simulink model "DataAnalysis"  (Simulink 7.6)
settings: Solver=FixedStepDiscrete  StartTime=0.0  StopTime=0  RelTol=1e-3
undefined symbols (not defined in the file or in its folder): gray, Rec, SDTV
libraries: vipconversions x2, vipsnks x1, viptextngfix x1, vipsrcs x1, viptransforms x1
settings Model: Creator=Administrator  LastModifiedBy=Administrator
settings OptimizationCC: OptimizeModelRefInitCode=on  LifeSpan=1
settings RTWCC: SystemTargetFile=ert.tlc  GenCodeOnly=on  TemplateMakefile=ert_default_tmf  Description=Real-Time Workshop Embedded Coder  GenerateReport=on  ProcessScript=ert_make_rtw_hook  IncludeHyperlinkInReport=on  LaunchReport=on  TargetLang=C++
settings CodeAppCC: IgnoreCustomStorageClasses=off
settings ERTTargetCC: MultiwordLength=2048  GenerateSampleERTMain=on  ERTCustomFileTemplate=example_file_process.tlc  ConvertIfToSwitch=off

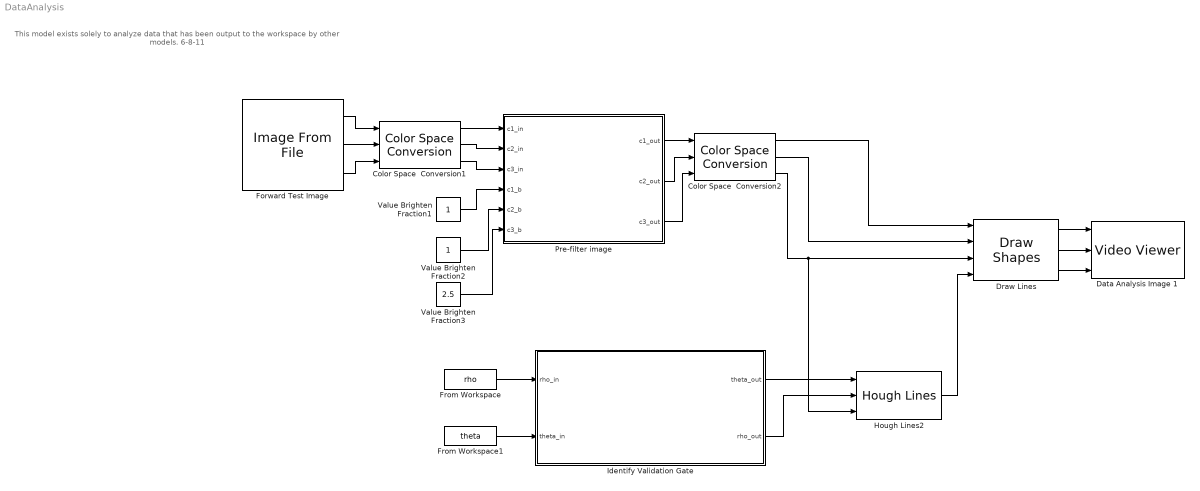
== system DataAnalysis ==
  note: This model exists solely to analyze
      | data that has been output to the
      | workspace by other models.
      |
      | 6-8-11
  Color Space  Conversion1 : vipconversions/Color Space  Conversion  conversion=Obsolete  conversionActive=R'G'B' to HSV  wp_str=D50  rec=Rec. 601 (SDTV)  sys=1125/60/2:1  imagePorts=Separate color signals
  Color Space  Conversion2 : vipconversions/Color Space  Conversion  conversion=Obsolete  conversionActive=HSV to R'G'B'  wp_str=D50  rec=Rec. 601 (SDTV)  sys=1125/60/2:1  imagePorts=Separate color signals
  Data Analysis Image 1 : vipsnks/Video Viewer  DialogControllerArgs=DataTag1  inputType=Obsolete7b  imagePorts=Separate color signals  useColorMap=off  colormapValue=gray(256)  specRange=off  minInputVal=0  maxInputVal=255  FigPos=[39 393 492 307]  AxisZoom=on  trueSizedOnce=off  OpenAtMdlStart=on
  Draw Lines : viptextngfix/Draw Shapes  DialogController=vipDDGCreate  DialogControllerArgs=DataTag2  shape=Lines  fill=off  fillClrSource=Specify via dialog  display=User-specified value  intensity=200  color=[.8 .8 .8]  opacity=0.6  viewport=Entire image  antialiasing=off  inType=Obsolete  imagePorts=Separate color signals  prodOutputMode=Binary point scaling  prodOutputWordLength=32  prodOutputFracLength=14  memoryMode=Specify word length  memoryWordLength=16  memoryFracLength=15  roundingMode=Floor  overflowMode=off
  Forward Test Image : vipsrcs/Image From File  Tag=vipblks_nd  DialogController=vipDDGCreate  DialogControllerArgs=DataTag3  SystemSampleTime=-1  FileName=C:\Documents and Settings\Administrator\My Documents\Academics\Summer 2011\AUVT\Models\Test_Models\Images\gate8.PNG  imagePorts=Separate color signals  Ts=-1  ImageDataType=double  Signed=on  WordLength=16  sdImageDataType=uint(8)  FractionLengthMode=User-defined  FractionLength=15  OutPortLabels=R|G|B
  From Workspace : FromWorkspace  VariableName=rho  SampleTime=0
  From Workspace1 : FromWorkspace  VariableName=theta  SampleTime=0
  Hough Lines2 : viptransforms/Hough Lines  DialogController=vipDDGCreate  DialogControllerArgs=DataTag4  sineCompMethod=Trigonometric function  thetaRes=pi/180  firstCoeffMode=Specify word length  firstCoeffWordLength=16  firstCoeffFracLength=15  prodOutputMode=Binary point scaling  prodOutputWordLength=32  prodOutputFracLength=16  roundingMode=Nearest  overflowMode=on
  Identify Validation Gate : Stateflow chart  TreatAsAtomicUnit=on  SystemSampleTime=[1/30 0]
  Pre-filter image : Stateflow chart  TreatAsAtomicUnit=on
  Value Brighten Fraction1 : Constant  SampleTime=-1
  Value Brighten Fraction2 : Constant  SampleTime=-1
  Value Brighten Fraction3 : Constant  Value=2.5  SampleTime=-1
  wires:
  Hough Lines2/1 -> Draw Lines/4
  Draw Lines/1 -> Data Analysis Image 1/1
  Draw Lines/2 -> Data Analysis Image 1/2
  Draw Lines/3 -> Data Analysis Image 1/3
  Identify Validation Gate/1(theta_out) -> Hough Lines2/1
  Identify Validation Gate/2(rho_out) -> Hough Lines2/2
  From Workspace/1 -> Identify Validation Gate/1(rho_in)
  From Workspace1/1 -> Identify Validation Gate/2(theta_in)
  Forward Test Image/1 -> Color Space  Conversion1/1
  Forward Test Image/2 -> Color Space  Conversion1/2
  Forward Test Image/3 -> Color Space  Conversion1/3
  Color Space  Conversion1/1 -> Pre-filter image/1(c1_in)
  Color Space  Conversion1/2 -> Pre-filter image/2(c2_in)
  Color Space  Conversion1/3 -> Pre-filter image/3(c3_in)
  Value Brighten Fraction1/1 -> Pre-filter image/4(c1_b)
  Value Brighten Fraction2/1 -> Pre-filter image/5(c2_b)
  Value Brighten Fraction3/1 -> Pre-filter image/6(c3_b)
  Pre-filter image/1(c1_out) -> Color Space  Conversion2/1
  Pre-filter image/2(c2_out) -> Color Space  Conversion2/2
  Pre-filter image/3(c3_out) -> Color Space  Conversion2/3
  Color Space  Conversion2/1 -> Draw Lines/1
  Color Space  Conversion2/2 -> Draw Lines/2
  Color Space  Conversion2/3 -> Draw Lines/3, Hough Lines2/3

== matlab function Identify Validation Gate ==
  data: rho_in input double; theta_out output double; rho_out output double; theta_in input double
function [theta_out, rho_out] = selectLines2View(rho_in, theta_in)
%#eml

nmax = 150;
offset = 0;

rho_out = double(zeros(1,nmax));
theta_out = double(zeros(1, nmax));

eps_theta = 15*pi/180;

for i = 1:nmax-1
    
    % Only store vertical and horizontal lines, within tolerance
    condition1 = ( abs(theta_in(i+offset) - pi/2 ) <= eps_theta || abs( theta_in(i+offset) + pi/2 ) <= eps_theta );
    condition2 = ( abs(theta_in(i+offset) - 0 ) <= eps_theta );
    if( condition1 || condition2)
        theta_out(i) = theta_in(i+offset);
        rho_out(i) = rho_in(i+offset);
    end
    
end

return

== matlab function Pre-filter image ==
  data: c1_in input double; c2_in input double; c3_in input double; c1_out output double; c2_out output double; c3_out output double; c1_b input double; c2_b input double; c3_b input double
function [c1_out, c2_out, c3_out] = brightenImage(c1_in, c2_in, c3_in, c1_b, c2_b, c3_b)
%#eml


if( c1_b < 0 )
    c1_out = -c1_b.*ones(size(c1_in));
else
    c1_out = c1_b.*c1_in;
end

if( c2_b < 0 )
    c2_out = -c2_b.*ones(size(c2_in));
else
    c2_out = c2_b.*c2_in;
end

if( c3_b < 0 )
    c3_out = -c3_b.*ones(size(c3_in));
else
    c3_out = c3_b.*c3_in;
end


return
